simulink model "rSFCL_GitHub_Sim"  (R2019a)
settings: Solver=VariableStepAuto  StartTime=0.0  StopTime=0.1  MaxStep=1e-5  RelTol=1e-6
values from neighbouring files (symbols this model uses):
  Coefficient_temperature = 0.47e-8    (= 4.7e-09)    [rSFCL_GitHub.m]
  Cond_thermique_YBCO = 8    [rSFCL_GitHub.m]
  Critere_champ_Elec = 100e-6    (= 0.0001)    [rSFCL_GitHub.m]
  Ep_module_Ag_Bas = Ep_Ag_Bas / Nbr_module_Ep_Ag_Bas    (= 1.8e-06)    [rSFCL_GitHub.m]
  Ep_module_Ag_Haut = Ep_Ag_Haut / Nbr_module_Ep_Ag_Haut    (= 2e-06)    [rSFCL_GitHub.m]
  Ep_module_Hast = Ep_Hast / Nbr_module_Ep_Hast    (= 0.0001)    [rSFCL_GitHub.m]
  Ep_module_YBCO = Ep_YBCO / Nbr_module_Ep_YBCO    (= 1e-06)    [rSFCL_GitHub.m]
  Jc_critique = 2.5e10    (= 25000000000)    [rSFCL_GitHub.m]
  Largeur_ruban = 4e-3    (= 0.004)    [rSFCL_GitHub.m]
  Longeur_module = Longueur_ruban_sain / Nombre_module_sain    (= 10)    [rSFCL_GitHub.m]
  MV_argent = 10490    [rSFCL_GitHub.m]
  MV_hast = 8890    [rSFCL_GitHub.m]
  MV_YBCO = 6410    [rSFCL_GitHub.m]
  n_supra = 15    [rSFCL_GitHub.m]
  Res_inter_sain = Rho_interface * Epaisseur_R_int / Surface_sain    (= 2.5e-10)    [rSFCL_GitHub.m]
  Resisitance_etat_normal = 30e-8    (= 3e-07)    [rSFCL_GitHub.m]
  Temp_azote_liquide = 77    [rSFCL_GitHub.m]
  Temp_critique_supra = 90    [rSFCL_GitHub.m]
libraries: fl_lib x146, nesl_utility x87, ee_lib x5
(part 1 of 2)
settings Model: Creator=gdidier  LastModifiedBy=gdidier
settings SolverCC: MaxConsecutiveZCs=1  MaxConsecutiveMinStep=10  ZeroCrossAlgorithm=Adaptive
settings DataIOCC: ReturnWorkspaceOutputs=off
settings DebuggingCC: IgnoredZcDiagnostic=none  ArithmeticOperatorsInVariantConditions=warning

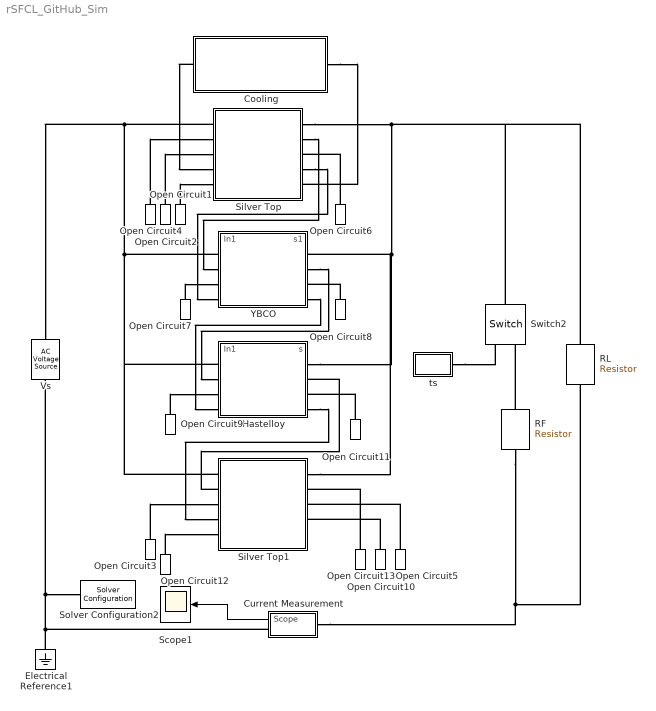
== system rSFCL_GitHub_Sim ==
  Cooling : Subsystem
  Current Measurement : Subsystem
  Electrical Reference1 : fl_lib/Electrical/Electrical Elements/Electrical Reference
  Hastelloy : Subsystem  mask{longueur=Longeur_module, largeur=Largeur_ruban, Ep_Hast=Ep_module_Hast, MV_Hast=MV_hast}
      mask prompts: longueur "Longueur ruban (m)"; largeur "Largeur ruban (m)"; Ep_Hast "Epaisseur hastelloy (m)"; MV_Hast "Masse volumique hastelloy (kg/m^3)"
      mask DialogControl DescGroupVar Prompt: Argent
      mask DialogControl DescTextVar Prompt: Limiteur de courant de court-circuit supraconducteur résistif
      mask Display:
      | port_label('output', 1, 'T_Hast')
      | port_label('input', 1, '')
      | %
      | port_label('lconn',1,'R_L')  %1
      | port_label('rconn',1, 'R_R') %2
      | %
      | port_label('lconn', 2, 'R_T')%3
      | port_label('rconn', 2, 'R_B') %4
      | %
      | port_label('lconn', 3, 'T_L') %5
      | port_label('rconn', 3, 'T_R') %6
      | %
      | port_label('lconn', 4, 'T_T') %7
      | port_label('rconn', 4, 'T_B') %8
      | %
      | color('red');disp('Hast')
  Open Circuit{1..13} (13 alike) : fl_lib/Electrical/Electrical Elements/Open Circuit  v_specify=off  v_priority=None  v=0 V  v_nominal_specify=off  v_nominal_unit=V  v_nominal_value=1
      settings: SourceProductName=Simscape  SourceProductBaseCode=SS
  RF : fl_lib/Electrical/Electrical Elements/Resistor  R=0.2631578947368421 Ohm  i_specify=off  i_priority=None  i=0 A  i_nominal_specify=off  i_nominal_unit=A  i_nominal_value=1  v_specify=off  v_priority=None  v=0 V  v_nominal_specify=off  v_nominal_unit=V  v_nominal_value=1
  RL : fl_lib/Electrical/Electrical Elements/Resistor  R=5 Ohm  i_specify=off  i_priority=None  i=0 A  i_nominal_specify=off  i_nominal_unit=A  i_nominal_value=1  v_specify=off  v_priority=None  v=0 V  v_nominal_specify=off  v_nominal_unit=V  v_nominal_value=1
  Scope1 : Scope
  Silver Top : Subsystem  mask{longueur=Longeur_module, largeur=Largeur_ruban, Ep_ar=Ep_module_Ag_Haut, MV_Ar=MV_argent}
      mask prompts: longueur "Longueur ruban (m)"; largeur "Largeur ruban (m)"; Ep_ar "Epaisseur argent (m)"; MV_Ar "Masse volumique argent (kg/m^3)"
      mask DialogControl DescGroupVar Prompt: Argent
      mask DialogControl DescTextVar Prompt: Limiteur de courant de court-circuit supraconducteur résistif
      mask Display:
      | %port_label('output', 1, 'T_I')
      | %port_label('input', 1, '')
      | %
      | %
      | port_label('lconn',1,'R_L')  %1
      | port_label('rconn',1, 'R_R') %2
      | %
      | port_label('lconn', 2, 'R_T')%3
      | port_label('rconn', 2, 'R_B') %4
      | %
      | port_label('lconn', 3, 'T_L') %5
      | port_label('rconn', 3, 'T_R') %6
      | %
      | port_label('lconn', 4, 'T_T') %7
      | port_label('rconn', 4, 'T_B') %8
      | %
      | port_label('rconn', 5, 'T_Silver_Top') %8
      | port_label('lconn', 5, 'ras') %9
      | 
      | %
      | color('red');disp('Silver')
  Silver Top1 : Subsystem  mask{longueur=Longeur_module, largeur=Largeur_ruban, Ep_ar=Ep_module_Ag_Bas, MV_Ar=MV_argent}
      mask prompts: longueur "Longueur ruban (m)"; largeur "Largeur ruban (m)"; Ep_ar "Epaisseur argent (m)"; MV_Ar "Masse volumique argent (kg/m^3)"
      mask DialogControl DescGroupVar Prompt: Argent
      mask DialogControl DescTextVar Prompt: Limiteur de courant de court-circuit supraconducteur résistif
      mask Display:
      | %port_label('output', 1, 'T_I')
      | %port_label('input', 1, '')
      | %
      | %
      | port_label('lconn',1,'R_L')  %1
      | port_label('rconn',1, 'R_R') %2
      | %
      | port_label('lconn', 2, 'R_T')%3
      | port_label('rconn', 2, 'R_B') %4
      | %
      | port_label('lconn', 3, 'T_L') %5
      | port_label('rconn', 3, 'T_R') %6
      | %
      | port_label('lconn', 4, 'T_T') %7
      | port_label('rconn', 4, 'T_B') %8
      | %
      | port_label('rconn', 5, 'T_Silver_Top') %8
      | port_label('lconn', 5, 'ras') %9
      | 
      | %
      | color('red');disp('Silver')
  Solver Configuration2 : nesl_utility/Solver Configuration  PhysicalDomain=network_engine_domain  SubClassName=solver  LeftPortType=input  RightPortType=generic  Tones=[]  Harmonics=[]  SimulateNoise=off  Profile=off  UseLocalSampling=off  EnableSwitchedLinearOptims=on  FrequencyDomain=off  UseCCode=off  RelTol=0.001  AbsTol=1e-06  MinStep=1e-09  ToWorkspace=off  RevertToSquareIcSolve=off  NumHomotopyIterations=100  PhasorMode=off  PhasorModeNumHarmonics=1  DoDC=off  ResidualTolerance=1e-09  UseLocalSolver=off  LocalSolverChoice=NE_BACKWARD_EULER_ADVANCER  LocalSolverSampleTime=0.001  DoFixedCost=off  MaxNonlinIter=3  MaxModeIter=2  LinearAlgebra=Sparse  EquationFormulation=NE_TIME_EF  DelaysMemoryBudget=1024  AutomaticFiltering=on  FilteringTimeConstant=0.001  PartitionStorageMethod=AS_NEEDED  PartitionMemoryBudget=1024  PartitionMethod=FAST
  Switch2 : fl_lib/Electrical/Electrical Elements/Switch  R_closed=0.000001 Ohm  G_open=1e-8 1/Ohm  Threshold=0.5  i_specify=off  i_priority=None  i=0 A  i_nominal_specify=off  i_nominal_unit=A  i_nominal_value=1  v_specify=off  v_priority=None  v=0 V  v_nominal_specify=off  v_nominal_unit=V  v_nominal_value=1
      settings: SourceProductName=Simscape
  Vs : fl_lib/Electrical/Electrical Sources/AC Voltage Source  amp=250 V  shift=0 deg  frequency=50 Hz  omega=0 rad/s
  "YBCO " : Subsystem  mask{longueur=Longeur_module, largeur=Largeur_ruban, Ep_YBCO=Ep_module_YBCO, MV_YBCO=MV_YBCO, k_YBCO=Cond_thermique_YBCO, Ec=Critere_champ_Elec, Tc=Temp_critique_supra, T0=Temp_azote_liquide, rho_Tc=Resisitance_etat_normal, a=Coefficient_temperature, Jc0=Jc_critique, n=n_supra}
      mask prompts: longueur "Longueur ruban (m)"; largeur "Largeur ruban (m)"; Ep_YBCO "Epaisseur YBCO (m)"; MV_YBCO "Masse volumique YBCO (kg/m^3)"; k_YBCO "Conductivité thermique YBCO (W/(K*m))"; Ec "Critère de champ électrique (V/m)"; Tc "Température critique supra (K)"; T0 "Température azote liquide (K)"; rho_Tc "Résistance à l'état normal (ohm*m)"; a "Coefficient de température (ohm*m/K)"; Jc0 "Densité de courant critique (A/m²)"; n "Exposant de la loi de puissance"
      mask DialogControl DescGroupVar Prompt: YBCO
      mask DialogControl DescTextVar Prompt: Limiteur de courant de court-circuit supraconducteur résistif
      mask Display:
      | port_label('output', 1, 'T_YBCO')
      | port_label('input', 1, '')
      | %
      | port_label('lconn',1,'R_L')  %1
      | port_label('rconn',1, 'R_R') %2
      | %
      | port_label('lconn', 2, 'R_T')%3
      | port_label('rconn', 2, 'R_B') %4
      | %
      | port_label('lconn', 3, 'T_L') %5
      | port_label('rconn', 3, 'T_R') %6
      | %
      | port_label('lconn', 4, 'T_T') %7
      | port_label('rconn', 4, 'T_B') %8
      | %
      | color('red');
      | 
      | disp('YBCO')
  ts : Subsystem
  wires:
  Current Measurement/1(Scope) -> Scope1/1
  connections:
  Silver Top/RConn1 -- RL/LConn1 -- Switch2/LConn1 -- Silver Top1/RConn1 -- Hastelloy/RConn1 -- "YBCO "/RConn1
  Electrical Reference1/LConn1 -- Current Measurement/RConn1 -- Vs/RConn1 -- Solver Configuration2/RConn1
  RF/RConn1 -- Current Measurement/LConn1 -- RL/RConn1
  RF/LConn1 -- Switch2/RConn2
  ts/RConn1 -- Switch2/RConn1
  Open Circuit1/LConn1 -- Silver Top/LConn5
  Cooling/RConn1 -- Silver Top/RConn5
  "YBCO "/RConn4 -- Hastelloy/LConn4
  Silver Top/LConn1 -- Vs/LConn1 -- Silver Top1/LConn1 -- Hastelloy/LConn1 -- "YBCO "/LConn1
  Silver Top/RConn2 -- "YBCO "/LConn2
  Silver Top/RConn4 -- "YBCO "/LConn4
  "YBCO "/RConn2 -- Hastelloy/LConn2
  Cooling/LConn1 -- Silver Top/LConn4
  Open Circuit2/LConn1 -- Silver Top/LConn3
  Open Circuit4/LConn1 -- Silver Top/LConn2
  Open Circuit6/LConn1 -- Silver Top/RConn3
  Open Circuit7/LConn1 -- "YBCO "/LConn3
  Open Circuit8/LConn1 -- "YBCO "/RConn3
  Open Circuit9/LConn1 -- Hastelloy/LConn3
  Open Circuit3/LConn1 -- Silver Top1/LConn3
  Open Circuit12/LConn1 -- Silver Top1/LConn5
  Hastelloy/RConn4 -- Silver Top1/LConn4
  Silver Top1/LConn2 -- Hastelloy/RConn2
  Open Circuit11/LConn1 -- Hastelloy/RConn3
  Open Circuit10/LConn1 -- Silver Top1/RConn4
  Open Circuit5/LConn1 -- Silver Top1/RConn3
  Open Circuit13/LConn1 -- Silver Top1/RConn2

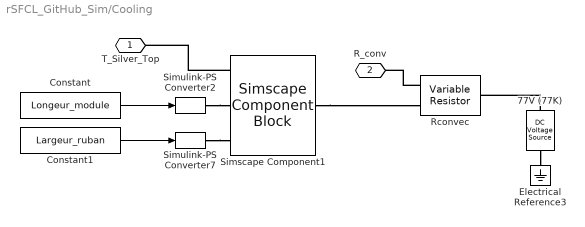
== system rSFCL_GitHub_Sim/Cooling ==
  77V (77K) : fl_lib/Electrical/Electrical Sources/DC Voltage Source  v0=77 V
  Constant : Constant  Value=Longeur_module
  Constant1 : Constant  Value=Largeur_ruban
  Electrical Reference3 : fl_lib/Electrical/Electrical Elements/Electrical Reference
  Rconvec : fl_lib/Electrical/Electrical Elements/Variable Resistor  Rmin=0 Ohm  i_specify=on  i_priority=None  i=500 A  i_nominal_specify=off  i_nominal_unit=A  i_nominal_value=1  v_specify=off  v_priority=None  v=0 V  v_nominal_specify=off  v_nominal_unit=V  v_nominal_value=1
  Simscape Component1 : SimscapeComponentBlock  SourceFile=Cooling  ComponentPath=Cooling  ComponentVariants=Cooling  ComponentVariantNames=Cooling  ClassName=Cooling  SchemaVersion=1
      settings: CopyFcn=simscape.engine.sli.internal.componentblockcallback(gcbh,'COPY')  PreCopyFcn=simscape.engine.sli.internal.componentblockcallback(gcbh,'PRECOPY')  PreDeleteFcn=simscape.engine.sli.internal.componentblockcallback(gcbh,'PREDELETE')
      mask Type: UseFunction1
  Simulink-PS Converter2 : nesl_utility/Simulink-PS Converter  PhysicalDomain=network_engine_domain  SubClassName=ps_input  LeftPortType=input  RightPortType=output  PseudoPeriodic=off  Frequencies=[]  NoiseDistribution=none  NoiseParameters=[]  Unit=1  AffineConversion=off  FilteringAndDerivatives=provide  SimscapeFilterOrder=1  InputFilterTimeConstant=0.001  UdotUserProvided=0
  Simulink-PS Converter7 : nesl_utility/Simulink-PS Converter  PhysicalDomain=network_engine_domain  SubClassName=ps_input  LeftPortType=input  RightPortType=output  PseudoPeriodic=off  Frequencies=[]  NoiseDistribution=none  NoiseParameters=[]  Unit=1  AffineConversion=off  FilteringAndDerivatives=provide  SimscapeFilterOrder=1  InputFilterTimeConstant=0.001  UdotUserProvided=0
  T_Silver_Top : PMIOPort  Side=Right
  R_conv : PMIOPort  Port=2  Side=Left
  wires:
  Constant/1 -> Simulink-PS Converter2/1
  Constant1/1 -> Simulink-PS Converter7/1
  connections:
  77V (77K)/RConn1 -- Electrical Reference3/LConn1
  77V (77K)/LConn1 -- Rconvec/RConn1
  Rconvec/LConn2 -- R_conv/RConn1
  Simulink-PS Converter7/RConn1 -- Simscape Component1/LConn3
  Simscape Component1/RConn1 -- Rconvec/LConn1
  Simscape Component1/LConn1 -- T_Silver_Top/RConn1
  Simulink-PS Converter2/RConn1 -- Simscape Component1/LConn2

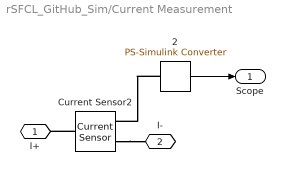
== system rSFCL_GitHub_Sim/Current Measurement ==
  "    2" : nesl_utility/PS-Simulink Converter  PhysicalDomain=network_engine_domain  SubClassName=ps_output  LeftPortType=input  RightPortType=output  PseudoPeriodic=off  Frequencies=[]  Unit=A  AffineConversion=off
  Current Sensor2 : fl_lib/Electrical/Electrical Sensors/Current Sensor
  I+ : PMIOPort  Side=Left
  I- : PMIOPort  Port=2  Side=Right
  Scope : Outport
  wires:
  "    2"/1 -> Scope/1
  connections:
  Current Sensor2/RConn2 -- I-/RConn1
  Current Sensor2/LConn1 -- I+/RConn1
  "    2"/LConn1 -- Current Sensor2/RConn1

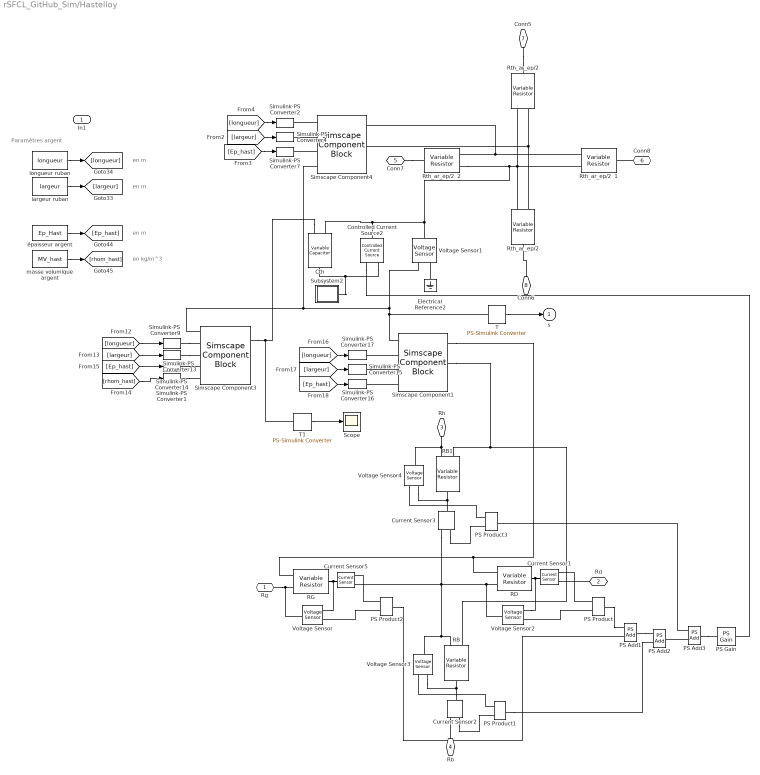
== system rSFCL_GitHub_Sim/Hastelloy ==
  note: en kg/m^3
  note: en m
  note: en m
  note: en m
  note: Paramètres argent
  In1 : Inport
  Controlled Current Source2 : fl_lib/Electrical/Electrical Sources/Controlled Current Source
  Cth : ee_lib/Passive/Variable Capacitor  prm=2  Cmin=1e-9 F  r=1e-6 Ohm  v0=0 V  q0=0 C
      settings: SourceProductName=Simscape Electrical  SourceProductBaseCode=PS
  Current Sensor{1..3,5} (4 alike) : fl_lib/Electrical/Electrical Sensors/Current Sensor
  Electrical Reference2 : fl_lib/Electrical/Electrical Elements/Electrical Reference
  PS Add1 : fl_lib/Physical Signals/Functions/PS Add
  PS Add2 : fl_lib/Physical Signals/Functions/PS Add
  PS Add3 : fl_lib/Physical Signals/Functions/PS Add
  PS Gain : fl_lib/Physical Signals/Functions/PS Gain  gain=1 1/V
  PS Product{,1..3} (4 alike) : fl_lib/Physical Signals/Functions/PS Product
      settings: SourceProductName=Simscape
  RB : fl_lib/Electrical/Electrical Elements/Variable Resistor  Rmin=RH Ohm  i_specify=off  i_priority=None  i=500 A  i_nominal_specify=off  i_nominal_unit=A  i_nominal_value=1  v_specify=off  v_priority=None  v=0 V  v_nominal_specify=off  v_nominal_unit=V  v_nominal_value=1
  RB1 : fl_lib/Electrical/Electrical Elements/Variable Resistor  Rmin=RH Ohm  i_specify=off  i_priority=None  i=500 A  i_nominal_specify=off  i_nominal_unit=A  i_nominal_value=1  v_specify=off  v_priority=None  v=0 V  v_nominal_specify=off  v_nominal_unit=V  v_nominal_value=1
  RD : fl_lib/Electrical/Electrical Elements/Variable Resistor  Rmin=RH Ohm  i_specify=off  i_priority=None  i=500 A  i_nominal_specify=off  i_nominal_unit=A  i_nominal_value=1  v_specify=off  v_priority=None  v=0 V  v_nominal_specify=off  v_nominal_unit=V  v_nominal_value=1
  RG : fl_lib/Electrical/Electrical Elements/Variable Resistor  Rmin=RH Ohm  i_specify=off  i_priority=None  i=500 A  i_nominal_specify=off  i_nominal_unit=A  i_nominal_value=1  v_specify=off  v_priority=None  v=0 V  v_nominal_specify=off  v_nominal_unit=V  v_nominal_value=1
  "Rth_ar_ep/2  " : fl_lib/Electrical/Electrical Elements/Variable Resistor  Rmin=RH Ohm  i_specify=off  i_priority=None  i=500 A  i_nominal_specify=off  i_nominal_unit=A  i_nominal_value=1  v_specify=off  v_priority=None  v=0 V  v_nominal_specify=off  v_nominal_unit=V  v_nominal_value=1
  "Rth_ar_ep/2    " : fl_lib/Electrical/Electrical Elements/Variable Resistor  Rmin=RH Ohm  i_specify=off  i_priority=None  i=500 A  i_nominal_specify=off  i_nominal_unit=A  i_nominal_value=1  v_specify=off  v_priority=None  v=0 V  v_nominal_specify=off  v_nominal_unit=V  v_nominal_value=1
  Rth_ar_ep/2  1 : fl_lib/Electrical/Electrical Elements/Variable Resistor  Rmin=RH Ohm  i_specify=off  i_priority=None  i=500 A  i_nominal_specify=off  i_nominal_unit=A  i_nominal_value=1  v_specify=off  v_priority=None  v=0 V  v_nominal_specify=off  v_nominal_unit=V  v_nominal_value=1
  Rth_ar_ep/2  2 : fl_lib/Electrical/Electrical Elements/Variable Resistor  Rmin=RH Ohm  i_specify=off  i_priority=None  i=500 A  i_nominal_specify=off  i_nominal_unit=A  i_nominal_value=1  v_specify=off  v_priority=None  v=0 V  v_nominal_specify=off  v_nominal_unit=V  v_nominal_value=1
  Scope : Scope
  Simscape Component1 : SimscapeComponentBlock  SourceFile=Res_Elec_Hast  ComponentPath=Res_Elec_Hast  ComponentVariants=Res_Elec_Hast  ComponentVariantNames=Res_Elec_Hast  ClassName=Res_Elec_Hast  SchemaVersion=1
      settings: CopyFcn=simscape.engine.sli.internal.componentblockcallback(gcbh,'COPY')  PreCopyFcn=simscape.engine.sli.internal.componentblockcallback(gcbh,'PRECOPY')  PreDeleteFcn=simscape.engine.sli.internal.componentblockcallback(gcbh,'PREDELETE')
      mask Type: UseFunction1
  Simscape Component3 : SimscapeComponentBlock  SourceFile=Cth_Hast  ComponentPath=Cth_Hast  ComponentVariants=Cth_Hast  ComponentVariantNames=Cth_Hast  ClassName=Cth_Hast  SchemaVersion=1
      settings: CopyFcn=simscape.engine.sli.internal.componentblockcallback(gcbh,'COPY')  PreCopyFcn=simscape.engine.sli.internal.componentblockcallback(gcbh,'PRECOPY')  PreDeleteFcn=simscape.engine.sli.internal.componentblockcallback(gcbh,'PREDELETE')
      mask Type: UseFunction1
  Simscape Component4 : SimscapeComponentBlock  SourceFile=Rth_Hast  ComponentPath=Rth_Hast  ComponentVariants=Rth_Hast  ComponentVariantNames=Rth_Hast  ClassName=Rth_Hast  SchemaVersion=1
      settings: CopyFcn=simscape.engine.sli.internal.componentblockcallback(gcbh,'COPY')  PreCopyFcn=simscape.engine.sli.internal.componentblockcallback(gcbh,'PRECOPY')  PreDeleteFcn=simscape.engine.sli.internal.componentblockcallback(gcbh,'PREDELETE')
      mask Type: UseFunction1
  Simulink-PS Converter{1..2,4,7,9,13..17} (10 alike) : nesl_utility/Simulink-PS Converter  PhysicalDomain=network_engine_domain  SubClassName=ps_input  LeftPortType=input  RightPortType=output  PseudoPeriodic=off  Frequencies=[]  NoiseDistribution=none  NoiseParameters=[]  Unit=1  AffineConversion=off  FilteringAndDerivatives=provide  SimscapeFilterOrder=1  InputFilterTimeConstant=0.001  UdotUserProvided=0
  Subsystem2 : Subsystem
  T : nesl_utility/PS-Simulink Converter  PhysicalDomain=network_engine_domain  SubClassName=ps_output  LeftPortType=input  RightPortType=output  PseudoPeriodic=off  Frequencies=[]  Unit=V  AffineConversion=off
  T1 : nesl_utility/PS-Simulink Converter  PhysicalDomain=network_engine_domain  SubClassName=ps_output  LeftPortType=input  RightPortType=output  PseudoPeriodic=off  Frequencies=[]  Unit=V  AffineConversion=off
  Voltage Sensor{,1..4} (5 alike) : fl_lib/Electrical/Electrical Sensors/Voltage Sensor
  largeur ruban : Constant  Value=largeur
  longueur ruban : Constant  Value=longueur
  masse volumique argent : Constant  Value=MV_hast
  épaisseur argent : Constant  Value=Ep_Hast
  Rg : PMIOPort  Side=Left
  Rd : PMIOPort  Port=2  Side=Right
  Rh : PMIOPort  Port=3  Side=Left
  Rb : PMIOPort  Port=4  Side=Right
  Conn7 : PMIOPort  Port=5  Side=Left
  Conn8 : PMIOPort  Port=6  Side=Right
  Conn5 : PMIOPort  Port=7  Side=Left
  Conn6 : PMIOPort  Port=8  Side=Right
  s : Outport
  wires:
  T/1 -> s/1
  longueur ruban/1 -> [longueur]
  épaisseur argent/1 -> [Ep_hast]
  masse volumique argent/1 -> [rhom_hast]
  largeur ruban/1 -> [largeur]
  [Ep_hast] -> Simulink-PS Converter14/1
  [largeur] -> Simulink-PS Converter13/1
  [rhom_hast] -> Simulink-PS Converter1/1
  [longueur] -> Simulink-PS Converter9/1
  [longueur] -> Simulink-PS Converter17/1
  [largeur] -> Simulink-PS Converter15/1
  [Ep_hast] -> Simulink-PS Converter16/1
  [Ep_hast] -> Simulink-PS Converter7/1
  [longueur] -> Simulink-PS Converter2/1
  [largeur] -> Simulink-PS Converter4/1
  T1/1 -> Scope/1
  connections:
  Current Sensor2/LConn1 -- Voltage Sensor3/RConn2 -- RB/RConn1
  Rth_ar_ep/2  1/LConn1 -- Simscape Component4/RConn1 -- Rth_ar_ep/2  2/LConn1
  RD/LConn1 -- Simscape Component1/RConn1 -- RG/LConn1
  RD/RConn1 -- Current Sensor1/LConn1 -- Voltage Sensor2/RConn2
  "Rth_ar_ep/2    "/LConn1 -- Simscape Component4/RConn2 -- "Rth_ar_ep/2  "/LConn1
  RG/RConn1 -- Current Sensor5/LConn1 -- Voltage Sensor/RConn2
  Subsystem2/LConn1 -- Cth/RConn1 -- Controlled Current Source2/RConn2
  Voltage Sensor/LConn1 -- RG/LConn2 -- Rg/RConn1
  Simscape Component3/LConn1 -- Simscape Component4/LConn4 -- Simscape Component1/LConn1 -- T/LConn1 -- Voltage Sensor1/RConn1
  PS Product1/LConn1 -- Voltage Sensor3/RConn1
  PS Product2/LConn2 -- Voltage Sensor/RConn1
  Rb/RConn1 -- Current Sensor2/RConn2
  Conn8/RConn1 -- Rth_ar_ep/2  1/RConn1
  Electrical Reference2/LConn1 -- Voltage Sensor1/RConn2
  PS Product/LConn1 -- Current Sensor1/RConn1
  PS Product2/LConn1 -- Current Sensor5/RConn1
  Conn7/RConn1 -- Rth_ar_ep/2  2/RConn1
  Current Sensor2/RConn1 -- PS Product1/LConn2
  Rd/RConn1 -- Current Sensor1/RConn2
  Simscape Component1/RConn2 -- RB1/LConn1 -- RB/LConn1
  PS Product/LConn2 -- Voltage Sensor2/RConn1
  PS Add1/RConn1 -- PS Add2/LConn1
  PS Product1/RConn1 -- PS Add2/LConn2
  PS Product/RConn1 -- PS Add1/LConn1
  PS Product2/RConn1 -- PS Add1/LConn2
  PS Add3/RConn1 -- PS Gain/LConn1
  Controlled Current Source2/RConn1 -- PS Gain/RConn1
  Cth/LConn1 -- Simscape Component3/RConn1 -- T1/LConn1
  Simscape Component4/LConn1 -- Simulink-PS Converter2/RConn1
  Simscape Component4/LConn2 -- Simulink-PS Converter4/RConn1
  Voltage Sensor4/RConn2 -- RB1/RConn1 -- Current Sensor3/LConn1
  RB1/LConn2 -- Voltage Sensor4/LConn1 -- Rh/RConn1
  PS Product3/LConn1 -- Voltage Sensor4/RConn1
  Current Sensor3/RConn1 -- PS Product3/LConn2
  PS Add3/LConn2 -- PS Add2/RConn1
  PS Add3/LConn1 -- PS Product3/RConn1
  Simulink-PS Converter13/RConn1 -- Simscape Component3/LConn3
  Simulink-PS Converter1/RConn1 -- Simscape Component3/LConn5
  Simulink-PS Converter14/RConn1 -- Simscape Component3/LConn4
  Simulink-PS Converter9/RConn1 -- Simscape Component3/LConn2
  Simscape Component1/LConn3 -- Simulink-PS Converter15/RConn1
  Simscape Component1/LConn4 -- Simulink-PS Converter16/RConn1
  Simscape Component1/LConn2 -- Simulink-PS Converter17/RConn1
  Simscape Component4/LConn3 -- Simulink-PS Converter7/RConn1
  RB/LConn2 -- Current Sensor5/RConn2 -- RD/LConn2 -- Voltage Sensor2/LConn1 -- Current Sensor3/RConn2 -- Voltage Sensor3/LConn1
  Conn5/RConn1 -- "Rth_ar_ep/2  "/RConn1
  Conn6/RConn1 -- "Rth_ar_ep/2    "/RConn1
  Controlled Current Source2/LConn1 -- Cth/LConn2 -- Voltage Sensor1/LConn1 -- Rth_ar_ep/2  2/LConn2 -- Rth_ar_ep/2  1/LConn2 -- "Rth_ar_ep/2    "/LConn2 -- "Rth_ar_ep/2  "/LConn2

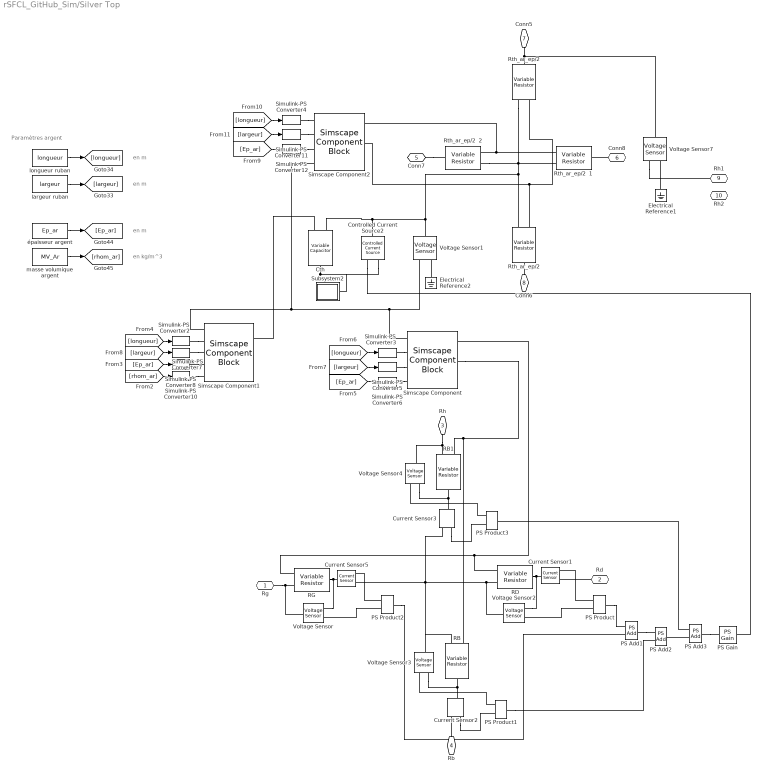
== system rSFCL_GitHub_Sim/Silver Top ==
  note: en kg/m^3
  note: en m
  note: en m
  note: en m
  note: Paramètres argent
  Controlled Current Source2 : fl_lib/Electrical/Electrical Sources/Controlled Current Source
  Cth : ee_lib/Passive/Variable Capacitor  prm=2  Cmin=1e-9 F  r=1e-6 Ohm  v0=0 V  q0=0 C
      settings: SourceProductName=Simscape Electrical  SourceProductBaseCode=PS
  Current Sensor{1..3,5} (4 alike) : fl_lib/Electrical/Electrical Sensors/Current Sensor
  Electrical Reference1 : fl_lib/Electrical/Electrical Elements/Electrical Reference
  Electrical Reference2 : fl_lib/Electrical/Electrical Elements/Electrical Reference
  PS Add1 : fl_lib/Physical Signals/Functions/PS Add
  PS Add2 : fl_lib/Physical Signals/Functions/PS Add
  PS Add3 : fl_lib/Physical Signals/Functions/PS Add
  PS Gain : fl_lib/Physical Signals/Functions/PS Gain  gain=1 1/V
  PS Product{,1..3} (4 alike) : fl_lib/Physical Signals/Functions/PS Product
      settings: SourceProductName=Simscape
  RB : fl_lib/Electrical/Electrical Elements/Variable Resistor  Rmin=Rag Ohm  i_specify=off  i_priority=None  i=500 A  i_nominal_specify=off  i_nominal_unit=A  i_nominal_value=1  v_specify=off  v_priority=None  v=0 V  v_nominal_specify=off  v_nominal_unit=V  v_nominal_value=1
  RB1 : fl_lib/Electrical/Electrical Elements/Variable Resistor  Rmin=Rag Ohm  i_specify=off  i_priority=None  i=500 A  i_nominal_specify=off  i_nominal_unit=A  i_nominal_value=1  v_specify=off  v_priority=None  v=0 V  v_nominal_specify=off  v_nominal_unit=V  v_nominal_value=1
  RD : fl_lib/Electrical/Electrical Elements/Variable Resistor  Rmin=Rag Ohm  i_specify=off  i_priority=None  i=500 A  i_nominal_specify=off  i_nominal_unit=A  i_nominal_value=1  v_specify=off  v_priority=None  v=0 V  v_nominal_specify=off  v_nominal_unit=V  v_nominal_value=1
  RG : fl_lib/Electrical/Electrical Elements/Variable Resistor  Rmin=Rag Ohm  i_specify=off  i_priority=None  i=500 A  i_nominal_specify=off  i_nominal_unit=A  i_nominal_value=1  v_specify=off  v_priority=None  v=0 V  v_nominal_specify=off  v_nominal_unit=V  v_nominal_value=1
  "Rth_ar_ep/2  " : fl_lib/Electrical/Electrical Elements/Variable Resistor  Rmin=Rag Ohm  i_specify=off  i_priority=None  i=500 A  i_nominal_specify=off  i_nominal_unit=A  i_nominal_value=1  v_specify=off  v_priority=None  v=0 V  v_nominal_specify=off  v_nominal_unit=V  v_nominal_value=1
  "Rth_ar_ep/2    " : fl_lib/Electrical/Electrical Elements/Variable Resistor  Rmin=Rag Ohm  i_specify=off  i_priority=None  i=500 A  i_nominal_specify=off  i_nominal_unit=A  i_nominal_value=1  v_specify=off  v_priority=None  v=0 V  v_nominal_specify=off  v_nominal_unit=V  v_nominal_value=1
  Rth_ar_ep/2  1 : fl_lib/Electrical/Electrical Elements/Variable Resistor  Rmin=Rag Ohm  i_specify=off  i_priority=None  i=500 A  i_nominal_specify=off  i_nominal_unit=A  i_nominal_value=1  v_specify=off  v_priority=None  v=0 V  v_nominal_specify=off  v_nominal_unit=V  v_nominal_value=1
  Rth_ar_ep/2  2 : fl_lib/Electrical/Electrical Elements/Variable Resistor  Rmin=Rag Ohm  i_specify=off  i_priority=None  i=500 A  i_nominal_specify=off  i_nominal_unit=A  i_nominal_value=1  v_specify=off  v_priority=None  v=0 V  v_nominal_specify=off  v_nominal_unit=V  v_nominal_value=1
  Simscape Component : SimscapeComponentBlock  SourceFile=Res_Elec_Ag  ComponentPath=Res_Elec_Ag  ComponentVariants=Res_Elec_Ag  ComponentVariantNames=Res_Elec_Ag  ClassName=Res_Elec_Ag  SchemaVersion=1
      settings: CopyFcn=simscape.engine.sli.internal.componentblockcallback(gcbh,'COPY')  PreCopyFcn=simscape.engine.sli.internal.componentblockcallback(gcbh,'PRECOPY')  PreDeleteFcn=simscape.engine.sli.internal.componentblockcallback(gcbh,'PREDELETE')
      mask Type: UseFunction1
  Simscape Component1 : SimscapeComponentBlock  SourceFile=Cth_Ag  ComponentPath=Cth_Ag  ComponentVariants=Cth_Ag  ComponentVariantNames=Cth_Ag  ClassName=Cth_Ag  SchemaVersion=1
      settings: CopyFcn=simscape.engine.sli.internal.componentblockcallback(gcbh,'COPY')  PreCopyFcn=simscape.engine.sli.internal.componentblockcallback(gcbh,'PRECOPY')  PreDeleteFcn=simscape.engine.sli.internal.componentblockcallback(gcbh,'PREDELETE')
      mask Type: UseFunction1
  Simscape Component2 : SimscapeComponentBlock  SourceFile=Rth_Ag  ComponentPath=Rth_Ag  ComponentVariants=Rth_Ag  ComponentVariantNames=Rth_Ag  ClassName=Rth_Ag  SchemaVersion=1
      settings: CopyFcn=simscape.engine.sli.internal.componentblockcallback(gcbh,'COPY')  PreCopyFcn=simscape.engine.sli.internal.componentblockcallback(gcbh,'PRECOPY')  PreDeleteFcn=simscape.engine.sli.internal.componentblockcallback(gcbh,'PREDELETE')
      mask Type: UseFunction1
  Simulink-PS Converter{2..8,10..12} (10 alike) : nesl_utility/Simulink-PS Converter  PhysicalDomain=network_engine_domain  SubClassName=ps_input  LeftPortType=input  RightPortType=output  PseudoPeriodic=off  Frequencies=[]  NoiseDistribution=none  NoiseParameters=[]  Unit=1  AffineConversion=off  FilteringAndDerivatives=provide  SimscapeFilterOrder=1  InputFilterTimeConstant=0.001  UdotUserProvided=0
  Subsystem2 : Subsystem
  Voltage Sensor{,1..4,7} (6 alike) : fl_lib/Electrical/Electrical Sensors/Voltage Sensor
  largeur ruban : Constant  Value=largeur
  longueur ruban : Constant  Value=longueur
  masse volumique argent : Constant  Value=MV_Ar
  épaisseur argent : Constant  Value=Ep_ar
  Rg : PMIOPort  Side=Left
  Rd : PMIOPort  Port=2  Side=Right
  Rh : PMIOPort  Port=3  Side=Left
  Rb : PMIOPort  Port=4  Side=Right
  Conn7 : PMIOPort  Port=5  Side=Left
  Conn8 : PMIOPort  Port=6  Side=Right
  Conn5 : PMIOPort  Port=7  Side=Left
  Conn6 : PMIOPort  Port=8  Side=Right
  Rh1 : PMIOPort  Port=9  Side=Right
  Rh2 : PMIOPort  Port=10  Side=Left
  wires:
  [largeur] -> Simulink-PS Converter5/1
  longueur ruban/1 -> [longueur]
  épaisseur argent/1 -> [Ep_ar]
  [longueur] -> Simulink-PS Converter3/1
  [Ep_ar] -> Simulink-PS Converter6/1
  masse volumique argent/1 -> [rhom_ar]
  largeur ruban/1 -> [largeur]
  [longueur] -> Simulink-PS Converter2/1
  [largeur] -> Simulink-PS Converter7/1
  [Ep_ar] -> Simulink-PS Converter8/1
  [rhom_ar] -> Simulink-PS Converter10/1
  [Ep_ar] -> Simulink-PS Converter12/1
  [longueur] -> Simulink-PS Converter4/1
  [largeur] -> Simulink-PS Converter11/1
  connections:
  Current Sensor2/LConn1 -- Voltage Sensor3/RConn2 -- RB/RConn1
  Rth_ar_ep/2  1/LConn1 -- Rth_ar_ep/2  2/LConn1 -- Simscape Component2/RConn1
  RG/LConn1 -- Simscape Component/RConn1 -- RD/LConn1
  Current Sensor1/LConn1 -- Voltage Sensor2/RConn2 -- RD/RConn1
  "Rth_ar_ep/2    "/LConn1 -- "Rth_ar_ep/2  "/LConn1 -- Simscape Component2/RConn2
  Current Sensor5/LConn1 -- Voltage Sensor/RConn2 -- RG/RConn1
  Cth/RConn1 -- Controlled Current Source2/RConn2 -- Subsystem2/LConn1
  RG/LConn2 -- Rg/RConn1 -- Voltage Sensor/LConn1
  Simscape Component1/LConn1 -- Simscape Component2/LConn4 -- Simscape Component/LConn1 -- Voltage Sensor1/RConn1
  Simulink-PS Converter6/RConn1 -- Simscape Component/LConn4
  Simulink-PS Converter3/RConn1 -- Simscape Component/LConn2
  PS Product1/LConn1 -- Voltage Sensor3/RConn1
  Electrical Reference1/LConn1 -- Voltage Sensor7/RConn2
  PS Product2/LConn2 -- Voltage Sensor/RConn1
  Rb/RConn1 -- Current Sensor2/RConn2
  Conn8/RConn1 -- Rth_ar_ep/2  1/RConn1
  Electrical Reference2/LConn1 -- Voltage Sensor1/RConn2
  Voltage Sensor7/RConn1 -- Rh1/RConn1
  PS Product/LConn1 -- Current Sensor1/RConn1
  PS Product2/LConn1 -- Current Sensor5/RConn1
  Conn7/RConn1 -- Rth_ar_ep/2  2/RConn1
  Current Sensor2/RConn1 -- PS Product1/LConn2
  Conn6/RConn1 -- "Rth_ar_ep/2    "/RConn1
  Rd/RConn1 -- Current Sensor1/RConn2
  Simscape Component/RConn2 -- RB1/LConn1 -- RB/LConn1
  Simulink-PS Converter5/RConn1 -- Simscape Component/LConn3
  PS Product/LConn2 -- Voltage Sensor2/RConn1
  PS Add1/RConn1 -- PS Add2/LConn1
  PS Product1/RConn1 -- PS Add2/LConn2
  PS Product/RConn1 -- PS Add1/LConn1
  PS Product2/RConn1 -- PS Add1/LConn2
  PS Add3/RConn1 -- PS Gain/LConn1
  Controlled Current Source2/RConn1 -- PS Gain/RConn1
  Simulink-PS Converter2/RConn1 -- Simscape Component1/LConn2
  Simulink-PS Converter7/RConn1 -- Simscape Component1/LConn3
  Simulink-PS Converter8/RConn1 -- Simscape Component1/LConn4
  Simulink-PS Converter10/RConn1 -- Simscape Component1/LConn5
  Cth/LConn1 -- Simscape Component1/RConn1
  Simulink-PS Converter4/RConn1 -- Simscape Component2/LConn1
  Simulink-PS Converter11/RConn1 -- Simscape Component2/LConn2
  Simulink-PS Converter12/RConn1 -- Simscape Component2/LConn3
  RB1/RConn1 -- Current Sensor3/LConn1 -- Voltage Sensor4/RConn2
  Voltage Sensor4/LConn1 -- Rh/RConn1 -- RB1/LConn2
  PS Product3/LConn1 -- Voltage Sensor4/RConn1
  Current Sensor3/RConn1 -- PS Product3/LConn2
  PS Add3/LConn2 -- PS Add2/RConn1
  PS Add3/LConn1 -- PS Product3/RConn1
  RD/LConn2 -- Current Sensor3/RConn2 -- Current Sensor5/RConn2 -- RB/LConn2 -- Voltage Sensor3/LConn1 -- Voltage Sensor2/LConn1
  Voltage Sensor7/LConn1 -- "Rth_ar_ep/2  "/RConn1 -- Conn5/RConn1
  Controlled Current Source2/LConn1 -- Cth/LConn2 -- Voltage Sensor1/LConn1 -- "Rth_ar_ep/2  "/LConn2 -- Rth_ar_ep/2  1/LConn2 -- Rth_ar_ep/2  2/LConn2 -- "Rth_ar_ep/2    "/LConn2

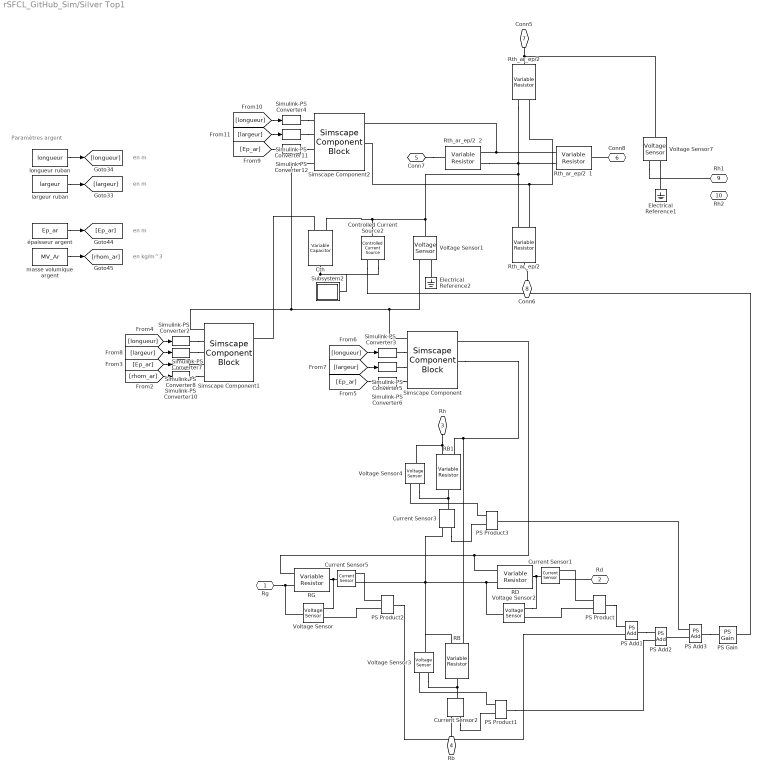
== system rSFCL_GitHub_Sim/Silver Top1 ==
  note: en kg/m^3
  note: en m
  note: en m
  note: en m
  note: Paramètres argent
  Controlled Current Source2 : fl_lib/Electrical/Electrical Sources/Controlled Current Source
  Cth : ee_lib/Passive/Variable Capacitor  prm=2  Cmin=1e-9 F  r=1e-6 Ohm  v0=0 V  q0=0 C
      settings: SourceProductName=Simscape Electrical  SourceProductBaseCode=PS
  Current Sensor{1..3,5} (4 alike) : fl_lib/Electrical/Electrical Sensors/Current Sensor
  Electrical Reference1 : fl_lib/Electrical/Electrical Elements/Electrical Reference
  Electrical Reference2 : fl_lib/Electrical/Electrical Elements/Electrical Reference
  PS Add1 : fl_lib/Physical Signals/Functions/PS Add
  PS Add2 : fl_lib/Physical Signals/Functions/PS Add
  PS Add3 : fl_lib/Physical Signals/Functions/PS Add
  PS Gain : fl_lib/Physical Signals/Functions/PS Gain  gain=1 1/V
  PS Product{,1..3} (4 alike) : fl_lib/Physical Signals/Functions/PS Product
      settings: SourceProductName=Simscape
  RB : fl_lib/Electrical/Electrical Elements/Variable Resistor  Rmin=Rag Ohm  i_specify=off  i_priority=None  i=500 A  i_nominal_specify=off  i_nominal_unit=A  i_nominal_value=1  v_specify=off  v_priority=None  v=0 V  v_nominal_specify=off  v_nominal_unit=V  v_nominal_value=1
  RB1 : fl_lib/Electrical/Electrical Elements/Variable Resistor  Rmin=Rag Ohm  i_specify=off  i_priority=None  i=500 A  i_nominal_specify=off  i_nominal_unit=A  i_nominal_value=1  v_specify=off  v_priority=None  v=0 V  v_nominal_specify=off  v_nominal_unit=V  v_nominal_value=1
  RD : fl_lib/Electrical/Electrical Elements/Variable Resistor  Rmin=Rag Ohm  i_specify=off  i_priority=None  i=500 A  i_nominal_specify=off  i_nominal_unit=A  i_nominal_value=1  v_specify=off  v_priority=None  v=0 V  v_nominal_specify=off  v_nominal_unit=V  v_nominal_value=1
  RG : fl_lib/Electrical/Electrical Elements/Variable Resistor  Rmin=Rag Ohm  i_specify=off  i_priority=None  i=500 A  i_nominal_specify=off  i_nominal_unit=A  i_nominal_value=1  v_specify=off  v_priority=None  v=0 V  v_nominal_specify=off  v_nominal_unit=V  v_nominal_value=1
  "Rth_ar_ep/2  " : fl_lib/Electrical/Electrical Elements/Variable Resistor  Rmin=Rag Ohm  i_specify=off  i_priority=None  i=500 A  i_nominal_specify=off  i_nominal_unit=A  i_nominal_value=1  v_specify=off  v_priority=None  v=0 V  v_nominal_specify=off  v_nominal_unit=V  v_nominal_value=1
  "Rth_ar_ep/2    " : fl_lib/Electrical/Electrical Elements/Variable Resistor  Rmin=Rag Ohm  i_specify=off  i_priority=None  i=500 A  i_nominal_specify=off  i_nominal_unit=A  i_nominal_value=1  v_specify=off  v_priority=None  v=0 V  v_nominal_specify=off  v_nominal_unit=V  v_nominal_value=1
  Rth_ar_ep/2  1 : fl_lib/Electrical/Electrical Elements/Variable Resistor  Rmin=Rag Ohm  i_specify=off  i_priority=None  i=500 A  i_nominal_specify=off  i_nominal_unit=A  i_nominal_value=1  v_specify=off  v_priority=None  v=0 V  v_nominal_specify=off  v_nominal_unit=V  v_nominal_value=1
  Rth_ar_ep/2  2 : fl_lib/Electrical/Electrical Elements/Variable Resistor  Rmin=Rag Ohm  i_specify=off  i_priority=None  i=500 A  i_nominal_specify=off  i_nominal_unit=A  i_nominal_value=1  v_specify=off  v_priority=None  v=0 V  v_nominal_specify=off  v_nominal_unit=V  v_nominal_value=1
  Simscape Component : SimscapeComponentBlock  SourceFile=Res_Elec_Ag  ComponentPath=Res_Elec_Ag  ComponentVariants=Res_Elec_Ag  ComponentVariantNames=Res_Elec_Ag  ClassName=Res_Elec_Ag  SchemaVersion=1
      settings: CopyFcn=simscape.engine.sli.internal.componentblockcallback(gcbh,'COPY')  PreCopyFcn=simscape.engine.sli.internal.componentblockcallback(gcbh,'PRECOPY')  PreDeleteFcn=simscape.engine.sli.internal.componentblockcallback(gcbh,'PREDELETE')
      mask Type: UseFunction1
  Simscape Component1 : SimscapeComponentBlock  SourceFile=Cth_Ag  ComponentPath=Cth_Ag  ComponentVariants=Cth_Ag  ComponentVariantNames=Cth_Ag  ClassName=Cth_Ag  SchemaVersion=1
      settings: CopyFcn=simscape.engine.sli.internal.componentblockcallback(gcbh,'COPY')  PreCopyFcn=simscape.engine.sli.internal.componentblockcallback(gcbh,'PRECOPY')  PreDeleteFcn=simscape.engine.sli.internal.componentblockcallback(gcbh,'PREDELETE')
      mask Type: UseFunction1
  Simscape Component2 : SimscapeComponentBlock  SourceFile=Rth_Ag  ComponentPath=Rth_Ag  ComponentVariants=Rth_Ag  ComponentVariantNames=Rth_Ag  ClassName=Rth_Ag  SchemaVersion=1
      settings: CopyFcn=simscape.engine.sli.internal.componentblockcallback(gcbh,'COPY')  PreCopyFcn=simscape.engine.sli.internal.componentblockcallback(gcbh,'PRECOPY')  PreDeleteFcn=simscape.engine.sli.internal.componentblockcallback(gcbh,'PREDELETE')
      mask Type: UseFunction1
  Simulink-PS Converter{2..8,10..12} (10 alike) : nesl_utility/Simulink-PS Converter  PhysicalDomain=network_engine_domain  SubClassName=ps_input  LeftPortType=input  RightPortType=output  PseudoPeriodic=off  Frequencies=[]  NoiseDistribution=none  NoiseParameters=[]  Unit=1  AffineConversion=off  FilteringAndDerivatives=provide  SimscapeFilterOrder=1  InputFilterTimeConstant=0.001  UdotUserProvided=0
  Subsystem2 : Subsystem
  Voltage Sensor{,1..4,7} (6 alike) : fl_lib/Electrical/Electrical Sensors/Voltage Sensor
  largeur ruban : Constant  Value=largeur
  longueur ruban : Constant  Value=longueur
  masse volumique argent : Constant  Value=MV_Ar
  épaisseur argent : Constant  Value=Ep_ar
  Rg : PMIOPort  Side=Left
  Rd : PMIOPort  Port=2  Side=Right
  Rh : PMIOPort  Port=3  Side=Left
  Rb : PMIOPort  Port=4  Side=Right
  Conn7 : PMIOPort  Port=5  Side=Left
  Conn8 : PMIOPort  Port=6  Side=Right
  Conn5 : PMIOPort  Port=7  Side=Left
  Conn6 : PMIOPort  Port=8  Side=Right
  Rh1 : PMIOPort  Port=9  Side=Right
  Rh2 : PMIOPort  Port=10  Side=Left
  wires:
  [largeur] -> Simulink-PS Converter5/1
  longueur ruban/1 -> [longueur]
  épaisseur argent/1 -> [Ep_ar]
  [longueur] -> Simulink-PS Converter3/1
  [Ep_ar] -> Simulink-PS Converter6/1
  masse volumique argent/1 -> [rhom_ar]
  largeur ruban/1 -> [largeur]
  [longueur] -> Simulink-PS Converter2/1
  [largeur] -> Simulink-PS Converter7/1
  [Ep_ar] -> Simulink-PS Converter8/1
  [rhom_ar] -> Simulink-PS Converter10/1
  [Ep_ar] -> Simulink-PS Converter12/1
  [longueur] -> Simulink-PS Converter4/1
  [largeur] -> Simulink-PS Converter11/1
  connections:
  Current Sensor2/LConn1 -- Voltage Sensor3/RConn2 -- RB/RConn1
  Rth_ar_ep/2  1/LConn1 -- Rth_ar_ep/2  2/LConn1 -- Simscape Component2/RConn1
  RG/LConn1 -- Simscape Component/RConn1 -- RD/LConn1
  Current Sensor1/LConn1 -- Voltage Sensor2/RConn2 -- RD/RConn1
  "Rth_ar_ep/2    "/LConn1 -- "Rth_ar_ep/2  "/LConn1 -- Simscape Component2/RConn2
  Current Sensor5/LConn1 -- Voltage Sensor/RConn2 -- RG/RConn1
  Cth/RConn1 -- Controlled Current Source2/RConn2 -- Subsystem2/LConn1
  RG/LConn2 -- Rg/RConn1 -- Voltage Sensor/LConn1
  Simscape Component1/LConn1 -- Simscape Component2/LConn4 -- Simscape Component/LConn1 -- Voltage Sensor1/RConn1
  Simulink-PS Converter6/RConn1 -- Simscape Component/LConn4
  Simulink-PS Converter3/RConn1 -- Simscape Component/LConn2
  PS Product1/LConn1 -- Voltage Sensor3/RConn1
  Electrical Reference1/LConn1 -- Voltage Sensor7/RConn2
  PS Product2/LConn2 -- Voltage Sensor/RConn1
  Rb/RConn1 -- Current Sensor2/RConn2
  Conn8/RConn1 -- Rth_ar_ep/2  1/RConn1
  Electrical Reference2/LConn1 -- Voltage Sensor1/RConn2
  Voltage Sensor7/RConn1 -- Rh1/RConn1
  PS Product/LConn1 -- Current Sensor1/RConn1
  PS Product2/LConn1 -- Current Sensor5/RConn1
  Conn7/RConn1 -- Rth_ar_ep/2  2/RConn1
  Current Sensor2/RConn1 -- PS Product1/LConn2
  Rd/RConn1 -- Current Sensor1/RConn2
  Simscape Component/RConn2 -- RB1/LConn1 -- RB/LConn1
  Simulink-PS Converter5/RConn1 -- Simscape Component/LConn3
  PS Product/LConn2 -- Voltage Sensor2/RConn1
  PS Add1/RConn1 -- PS Add2/LConn1
  PS Product1/RConn1 -- PS Add2/LConn2
  PS Product/RConn1 -- PS Add1/LConn1
  PS Product2/RConn1 -- PS Add1/LConn2
  PS Add3/RConn1 -- PS Gain/LConn1
  Controlled Current Source2/RConn1 -- PS Gain/RConn1
  Simulink-PS Converter2/RConn1 -- Simscape Component1/LConn2
  Simulink-PS Converter7/RConn1 -- Simscape Component1/LConn3
  Simulink-PS Converter8/RConn1 -- Simscape Component1/LConn4
  Simulink-PS Converter10/RConn1 -- Simscape Component1/LConn5
  Cth/LConn1 -- Simscape Component1/RConn1
  Simulink-PS Converter4/RConn1 -- Simscape Component2/LConn1
  Simulink-PS Converter11/RConn1 -- Simscape Component2/LConn2
  Simulink-PS Converter12/RConn1 -- Simscape Component2/LConn3
  RB1/RConn1 -- Current Sensor3/LConn1 -- Voltage Sensor4/RConn2
  Voltage Sensor4/LConn1 -- Rh/RConn1 -- RB1/LConn2
  PS Product3/LConn1 -- Voltage Sensor4/RConn1
  Current Sensor3/RConn1 -- PS Product3/LConn2
  PS Add3/LConn2 -- PS Add2/RConn1
  PS Add3/LConn1 -- PS Product3/RConn1
  RD/LConn2 -- Current Sensor3/RConn2 -- Current Sensor5/RConn2 -- RB/LConn2 -- Voltage Sensor3/LConn1 -- Voltage Sensor2/LConn1
  Voltage Sensor7/LConn1 -- "Rth_ar_ep/2  "/RConn1 -- Conn5/RConn1
  Controlled Current Source2/LConn1 -- Cth/LConn2 -- Voltage Sensor1/LConn1 -- "Rth_ar_ep/2  "/LConn2 -- Rth_ar_ep/2  1/LConn2 -- Rth_ar_ep/2  2/LConn2 -- "Rth_ar_ep/2    "/LConn2
  Conn6/RConn1 -- "Rth_ar_ep/2    "/RConn1
